simulink model "simulinkblocks"  (R2025b)
settings: Solver=FixedStepAuto  StartTime=0.0  StopTime=10.0  RelTol=1e-3  EnableMultiTasking=on
libraries: arduinolib x18, simulink x3
settings Model: ExtModeTrigDuration=2  Creator=jenis  LastModifiedBy=jenis
settings SolverCC: AutoInsertRateTranBlk=on
settings OptimizationCC: EnhancedBackFolding=on  PassReuseOutputArgsAs=Individual arguments  ZeroExternalMemoryAtStartup=off  ZeroInternalMemoryAtStartup=off  MaxStackSize=64  OptimizeBlockOrder=speed  DifferentSizesBufferReuse=on  OptimizationCustomize=off  EfficientTunableParamExpr=on
settings DebuggingCC: ParameterTunabilityLossMsg=error
settings HardwareCC: ProdBitPerInt=16.0  ProdBitPerPointer=16.0  ProdBitPerSizeT=16.0  ProdBitPerPtrDiffT=16.0  ProdLargestAtomicFloat=None  ProdWordSize=8.0  ProdHWDeviceType=Atmel->AVR  UseEmbeddedCoderFeatures=off  UseSimulinkCoderFeatures=off
settings SFSimCC: MATLABDynamicMemAlloc=off
settings RTWCC: SystemTargetFile=ert.tlc  HardwareBoard=Arduino Uno  TemplateMakefile=ert_default_tmf  Toolchain=Arduino AVR  BuildConfiguration=Faster Runs  Description=Embedded Coder
settings CodeAppCC: ForceParamTrailComments=on  IgnoreCustomStorageClasses=off  OperatorAnnotations=on  SimulinkDataObjDesc=on  SFDataObjDesc=on  InsertBlockDesc=on
settings ERTTargetCC: ExtModeTransport=3.0  ExtModeStaticAlloc=on  ExtModeAutomaticAllocSize=off  ExtModeStaticAllocSize=250.0  ExtModeMexFile=ext_xcp  ExtModeIntrfLevel=Level2 - Open  InlinedParameterPlacement=Hierarchical  SupportContinuousTime=on  SupportNonInlinedSFcns=on  SupportVariableSizeSignals=on

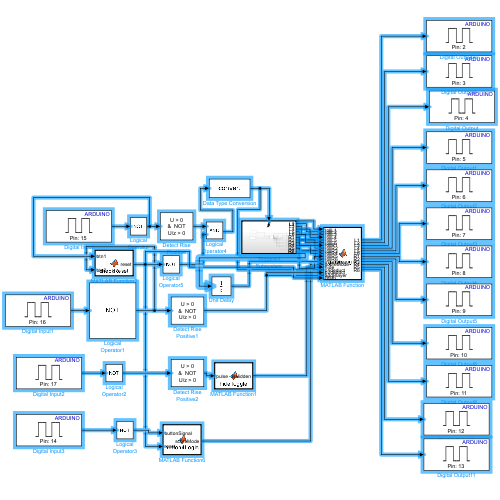
[thumbnail: Simulink's stored preview of the top-level diagram]
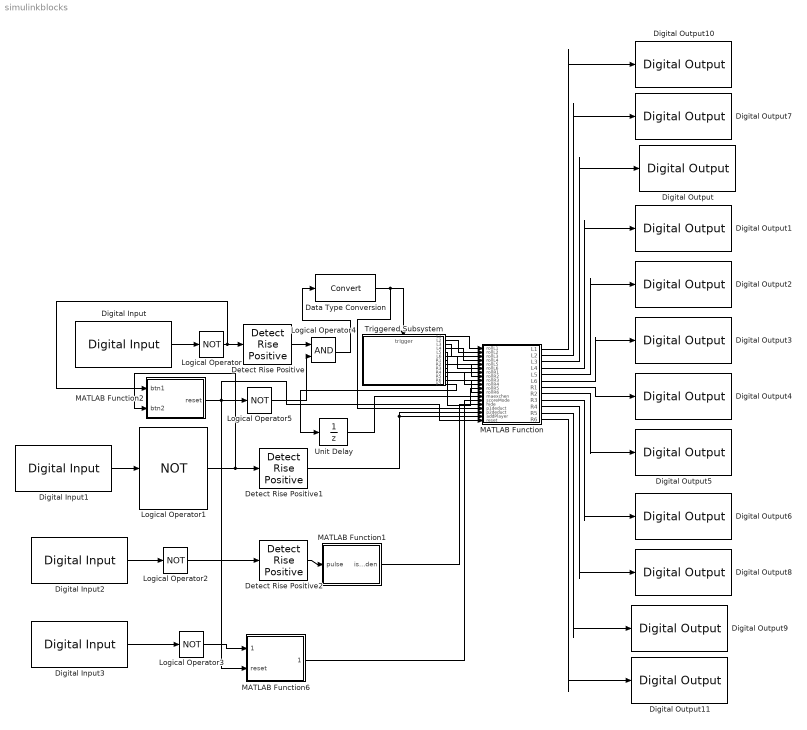
== system simulinkblocks ==
  Data Type Conversion : DataTypeConversion  SaturateOnIntegerOverflow=off  RndMeth=Floor
  Detect Rise Positive : simulink/Logic and Bit Operations/Detect Rise Positive  vinit=0  OutDataTypeStr=uint8
  Detect Rise Positive1 : simulink/Logic and Bit Operations/Detect Rise Positive  vinit=0  OutDataTypeStr=uint8
  Detect Rise Positive2 : simulink/Logic and Bit Operations/Detect Rise Positive  vinit=1  OutDataTypeStr=uint8
  Digital Input : arduinolib/Digital Input  pinNumber=15  mode=Input Pullup  Direction=input  SampleTime=0.1  blockPlatform=arduino
  Digital Input1 : arduinolib/Digital Input  pinNumber=16  mode=Input Pullup  Direction=input  SampleTime=0.1  blockPlatform=arduino
  Digital Input2 : arduinolib/Digital Input  pinNumber=17  mode=Input Pullup  Direction=input  SampleTime=0.1  blockPlatform=arduino
  Digital Input3 : arduinolib/Digital Input  pinNumber=14  mode=Input Pullup  Direction=input  SampleTime=0.1  blockPlatform=arduino
  Digital Output : arduinolib/Digital Output  pinNumber=4  Direction=output  blockPlatform=arduino
  Digital Output1 : arduinolib/Digital Output  pinNumber=5  Direction=output  blockPlatform=arduino
  Digital Output10 : arduinolib/Digital Output  pinNumber=2  Direction=output  blockPlatform=arduino
  Digital Output11 : arduinolib/Digital Output  pinNumber=13  Direction=output  blockPlatform=arduino
  Digital Output2 : arduinolib/Digital Output  pinNumber=6  Direction=output  blockPlatform=arduino
  Digital Output3 : arduinolib/Digital Output  pinNumber=7  Direction=output  blockPlatform=arduino
  Digital Output4 : arduinolib/Digital Output  pinNumber=8  Direction=output  blockPlatform=arduino
  Digital Output5 : arduinolib/Digital Output  pinNumber=9  Direction=output  blockPlatform=arduino
  Digital Output6 : arduinolib/Digital Output  pinNumber=10  Direction=output  blockPlatform=arduino
  Digital Output7 : arduinolib/Digital Output  pinNumber=3  Direction=output  blockPlatform=arduino
  Digital Output8 : arduinolib/Digital Output  pinNumber=11  Direction=output  blockPlatform=arduino
  Digital Output9 : arduinolib/Digital Output  pinNumber=12  Direction=output  blockPlatform=arduino
  Logical Operator{,1..3,5} (5 alike) : Logic  Operator=NOT  AllPortsSameDT=off  OutDataTypeStr=boolean
  Logical Operator4 : Logic  AllPortsSameDT=off  OutDataTypeStr=boolean
  MATLAB Function : MATLAB Function  TreatAsAtomicUnit=on
  MATLAB Function1 : MATLAB Function  TreatAsAtomicUnit=on
  MATLAB Function2 : MATLAB Function  TreatAsAtomicUnit=on
  MATLAB Function6 : MATLAB Function  TreatAsAtomicUnit=on
  Triggered Subsystem : Subsystem  TreatAsAtomicUnit=on
  Unit Delay : UnitDelay  SampleTime=0.1  HasFrameUpgradeWarning=on
  wires:
  Digital Input/1 -> Logical Operator/1
  Data Type Conversion/1 -> MATLAB Function/16(p1deduct), Triggered Subsystem/Trigger
  MATLAB Function/12(R6) -> Digital Output11/1
  Logical Operator4/1 -> Data Type Conversion/1
  MATLAB Function/6(L6) -> Digital Output3/1
  Triggered Subsystem/5(L5) -> MATLAB Function/5(rollL5)
  MATLAB Function/2(L2) -> Digital Output7/1
  Triggered Subsystem/2(L2) -> MATLAB Function/2(rollL2)
  Digital Input1/1 -> Logical Operator1/1
  Logical Operator5/1 -> Logical Operator4/2
  Triggered Subsystem/1(L1) -> MATLAB Function/1(rollL1)
  Triggered Subsystem/8(R2) -> MATLAB Function/8(rollR2)
  Digital Input2/1 -> Logical Operator2/1
  MATLAB Function/11(R5) -> Digital Output9/1
  Unit Delay/1 -> MATLAB Function/13(maexchen)
  Logical Operator2/1 -> Detect Rise Positive2/1
  MATLAB Function/7(R1) -> Digital Output4/1
  MATLAB Function/5(L5) -> Digital Output2/1
  Triggered Subsystem/3(L3) -> MATLAB Function/3(rollL3)
  MATLAB Function6/1(scoreMode) -> MATLAB Function/14(scoreMode)
  Logical Operator/1 -> Detect Rise Positive/1, MATLAB Function2/1(btn1)
  Triggered Subsystem/12(R6) -> MATLAB Function/12(rollR6)
  Detect Rise Positive/1 -> Logical Operator4/1
  MATLAB Function/8(R2) -> Digital Output5/1
  Digital Input3/1 -> Logical Operator3/1
  MATLAB Function1/1(isHidden) -> MATLAB Function/15(hide)
  Detect Rise Positive1/1 -> MATLAB Function/17(p2deduct), MATLAB Function/18(addPlayer)
  Logical Operator1/1 -> MATLAB Function2/2(btn2), Detect Rise Positive1/1
  Logical Operator3/1 -> MATLAB Function6/1(buttonSignal)
  MATLAB Function/1(L1) -> Digital Output10/1
  Triggered Subsystem/4(L4) -> MATLAB Function/4(rollL4)
  Triggered Subsystem/9(R3) -> MATLAB Function/9(rollR3)
  MATLAB Function/4(L4) -> Digital Output1/1
  MATLAB Function2/1(reset) -> MATLAB Function6/2(reset), MATLAB Function/19(reset), Logical Operator5/1
  Triggered Subsystem/6(L6) -> MATLAB Function/6(rollL6)
  Triggered Subsystem/10(R4) -> MATLAB Function/10(rollR4)
  MATLAB Function/9(R3) -> Digital Output6/1
  Triggered Subsystem/7(R1) -> MATLAB Function/7(rollR1)
  Detect Rise Positive2/1 -> MATLAB Function1/1(pulse)
  MATLAB Function/3(L3) -> Digital Output/1
  Triggered Subsystem/11(R5) -> MATLAB Function/11(rollR5)
  MATLAB Function/10(R4) -> Digital Output8/1
  Triggered Subsystem/13(R7) -> Unit Delay/1

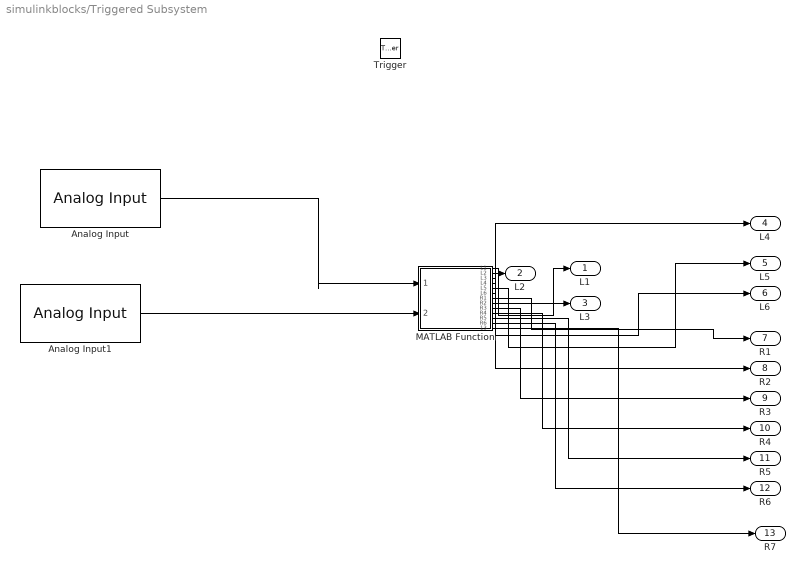
== system simulinkblocks/Triggered Subsystem ==
  Trigger : TriggerPort  VariantControl=(inherit)
  Analog Input : arduinolib/Analog Input  pinNumber=4  ReadResultsOnly=off  ConversionTriggerSource=Software  ExternalTriggerType=uint32( 0 )  OutputDataType=uint16  EnableConversionCompleteNotify=off  EnableOuputStatus=off  SampleTime=-1  blockPlatform=arduino
  Analog Input1 : arduinolib/Analog Input  pinNumber=5  ReadResultsOnly=off  ConversionTriggerSource=Software  ExternalTriggerType=uint32( 0 )  OutputDataType=uint16  EnableConversionCompleteNotify=off  EnableOuputStatus=off  SampleTime=-1  blockPlatform=arduino
  MATLAB Function : MATLAB Function  TreatAsAtomicUnit=on
  L1 : Outport
  L2 : Outport  Port=2
  L3 : Outport  Port=3
  L4 : Outport  Port=4
  L5 : Outport  Port=5
  L6 : Outport  Port=6
  R1 : Outport  Port=7
  R2 : Outport  Port=8
  R3 : Outport  Port=9
  R4 : Outport  Port=10
  R5 : Outport  Port=11
  R6 : Outport  Port=12
  R7 : Outport  Port=13
  wires:
  Analog Input/1 -> MATLAB Function/1(antenna1)
  Analog Input1/1 -> MATLAB Function/2(antenna2)
  MATLAB Function/1(L1) -> L1/1
  MATLAB Function/2(L2) -> L2/1
  MATLAB Function/3(L3) -> L3/1
  MATLAB Function/4(L4) -> L4/1
  MATLAB Function/5(L5) -> L5/1
  MATLAB Function/6(L6) -> L6/1
  MATLAB Function/7(R1) -> R1/1
  MATLAB Function/8(R2) -> R2/1
  MATLAB Function/9(R3) -> R3/1
  MATLAB Function/10(R4) -> R4/1
  MATLAB Function/11(R5) -> R5/1
  MATLAB Function/12(R6) -> R6/1
  MATLAB Function/13(maexchen) -> R7/1

== matlab function simulinkblocks/MATLAB Function2 ==
  data: btn1 input; reset output; btn2 input
function reset = checkReset(btn1, btn2)
    persistent holdCount;
    if isempty(holdCount)
        holdCount = uint8(0);
    end
    
    reset = uint8(0);
    
    if uint8(btn1) == uint8(1) && uint8(btn2) == uint8(1)
        holdCount = holdCount + uint8(1);
        if holdCount >= uint8(3)
            reset = uint8(1);
        end
    else
        holdCount = uint8(0);
    end
end

== matlab function simulinkblocks/MATLAB Function6 ==
  data: scoreMode output; buttonSignal input; reset input
function scoreMode = button4Logic(buttonSignal, reset)
    persistent pressCount isScore;
    if isempty(pressCount)
        pressCount = uint8(0);
        isScore = uint8(0);
    end
    
    if uint8(reset) == uint8(1)
        isScore = uint8(0);
    end
    
    if uint8(buttonSignal) == uint8(1)
        pressCount = pressCount + uint8(1);
    else
        if pressCount > uint8(0)
            if isScore == uint8(0)
                isScore = uint8(1);
            else
                isScore = uint8(0);
            end
        end
        pressCount = uint8(0);
    end
    
    scoreMode = isScore;
end

== matlab function simulinkblocks/MATLAB Function ==
  data: rollL1 input; L1 output; rollL2 input; rollL3 input; rollL4 input; rollL5 input; rollL6 input; rollR1 input; rollR2 input; rollR3 input; rollR4 input; rollR5 input; rollR6 input; maexchen input; scoreMode input; hide input; p1deduct input; p2deduct input; L2 output; L3 output; L4 output; L5 output; L6 output; R1 output; R2 output; R3 output; R4 output; R5 output; R6 output; addPlayer input; reset input
function [L1,L2,L3,L4,L5,L6,R1,R2,R3,R4,R5,R6] = gameLogic(rollL1,rollL2,rollL3,rollL4,rollL5,rollL6,rollR1,rollR2,rollR3,rollR4,rollR5,rollR6,maexchen,scoreMode,hide,p1deduct,p2deduct,addPlayer,reset)
    persistent p1life p2life flashCount state playerCount lockout;
    if isempty(state)
        p1life = uint8(6);
        p2life = uint8(6);
        flashCount = uint8(0);
        state = uint8(0);
        playerCount = uint8(2);
        lockout = uint8(0);
    end
    if uint8(reset) == uint8(1)
        state = uint8(0);
        p1life = uint8(6);
        p2life = uint8(6);
        playerCount = uint8(2);
        flashCount = uint8(0);
        lockout = uint8(20);
    end
    if lockout > uint8(0)
        lockout = lockout - uint8(1);
    end
    if state == uint8(0)
        if addPlayer == 1
            playerCount = playerCount + uint8(1);
            if playerCount > uint8(6)
                playerCount = uint8(2);
            end
        end
        if (rollL1 == 1 || rollR1 == 1) && lockout == uint8(0)
            state = uint8(1);
        end
    end
    if state == uint8(1)
        if p1deduct == 1 && scoreMode == 1 && p1life > uint8(0)
            p1life = p1life - uint8(1);
        end
        if p2deduct == 1 && scoreMode == 1 && p2life > uint8(0)
            p2life = p2life - uint8(1);
        end
        if maexchen == 1 || p1life == uint8(0) || p2life == uint8(0)
            state = uint8(2);
            flashCount = uint8(40);
        end
    end
    if state == uint8(2)
        if flashCount > uint8(0)
            flashCount = flashCount - uint8(1);
        else
            state = uint8(0);
            p1life = uint8(6);
            p2life = uint8(6);
            playerCount = uint8(2);
            lockout = uint8(20);
        end
    end
    if state == uint8(2)
        if mod(flashCount, uint8(2)) == uint8(0)
            L1=uint8(1); L2=uint8(1); L3=uint8(1);
            L4=uint8(1); L5=uint8(1); L6=uint8(1);
            R1=uint8(1); R2=uint8(1); R3=uint8(1);
            R4=uint8(1); R5=uint8(1); R6=uint8(1);
        else
            L1=uint8(0); L2=uint8(0); L3=uint8(0);
            L4=uint8(0); L5=uint8(0); L6=uint8(0);
            R1=uint8(0); R2=uint8(0); R3=uint8(0);
            R4=uint8(0); R5=uint8(0); R6=uint8(0);
        end
    elseif state == uint8(0)
        L1=uint8(playerCount>=1); L2=uint8(playerCount>=2);
        L3=uint8(playerCount>=3); L4=uint8(playerCount>=4);
        L5=uint8(playerCount>=5); L6=uint8(playerCount>=6);
        R1=uint8(0); R2=uint8(0); R3=uint8(0);
        R4=uint8(0); R5=uint8(0); R6=uint8(0);
    elseif scoreMode == 1 && state == uint8(1)
        L1=uint8(p1life>=1); L2=uint8(p1life>=2); L3=uint8(p1life>=3);
        L4=uint8(p1life>=4); L5=uint8(p1life>=5); L6=uint8(p1life>=6);
        R1=uint8(p2life>=1); R2=uint8(p2life>=2); R3=uint8(p2life>=3);
        R4=uint8(p2life>=4); R5=uint8(p2life>=5); R6=uint8(p2life>=6);
    elseif hide == 1
        L1=uint8(0); L2=uint8(0); L3=uint8(0);
        L4=uint8(0); L5=uint8(0); L6=uint8(0);
        R1=uint8(0); R2=uint8(0); R3=uint8(0);
        R4=uint8(0); R5=uint8(0); R6=uint8(0);
    else
        L1=rollL1; L2=rollL2; L3=rollL3;
        L4=rollL4; L5=rollL5; L6=rollL6;
        R1=rollR1; R2=rollR2; R3=rollR3;
        R4=rollR4; R5=rollR5; R6=rollR6;
    end
end

== matlab function simulinkblocks/Triggered Subsystem/MATLAB Function ==
  data: antenna1 input; L1 output; antenna2 input; L2 output; L3 output; L4 output; L5 output; L6 output; R1 output; R2 output; R3 output; R4 output; R5 output; R6 output; maexchen output
function [L1,L2,L3,L4,L5,L6,R1,R2,R3,R4,R5,R6,maexchen] = rollTwoDice(antenna1, antenna2)
    rollA = uint8(mod(antenna1 * 173, 6) + 1);
    rollB = uint8(mod(antenna2 * 137, 6) + 1);
    if rollA >= rollB
        high = rollA; low = rollB;
    else
        high = rollB; low = rollA;
    end
    L1=uint8(high>=1); L2=uint8(high>=2); L3=uint8(high>=3);
    L4=uint8(high>=4); L5=uint8(high>=5); L6=uint8(high==6);
    R1=uint8(low>=1);  R2=uint8(low>=2);  R3=uint8(low>=3);
    R4=uint8(low>=4);  R5=uint8(low>=5);  R6=uint8(low==6);
    if high == uint8(2) && low == uint8(1)
        maexchen = uint8(1);
    else
        maexchen = uint8(0);
    end
end

== matlab function simulinkblocks/MATLAB Function1 ==
  data: pulse input; isHidden output
function isHidden = hideToggle(pulse)
    persistent state;
    if isempty(state)
        state = uint8(0);
    end
    
    if pulse == uint8(1)
        if state == uint8(0)
            state = uint8(1);
        else
            state = uint8(0);
        end
    end
    
    isHidden = state;
end
